simulink model "control_motor"  (R2025a)
settings: Solver=VariableStepAuto  StartTime=0.0  StopTime=10.0  RelTol=1e-3
libraries: fuzblock x1
settings Model: Creator=Bremdows  LastModifiedBy=Bremdows

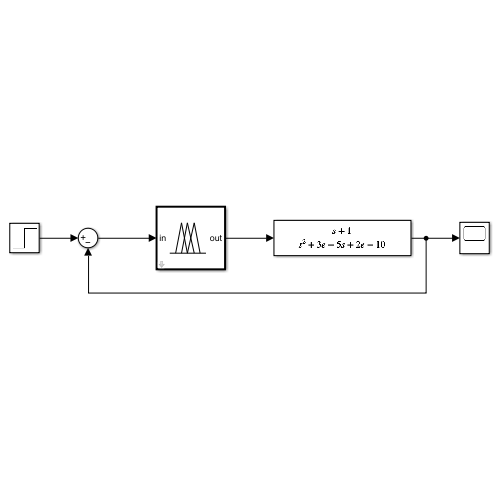
[thumbnail: Simulink's stored preview of the top-level diagram]
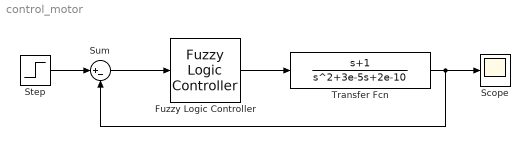
== system control_motor ==
  Fuzzy Logic Controller : fuzblock/Fuzzy Logic  Controller  FIS=faja_motor  OutputSampleNumber=101  DataType=double  UseLookupTable=off  NumBreakpoints=10  FuzzifiedInputs=off  RuleFiringStrengths=off  RuleOutputs=off  AggregatedOutputs=off  SimulateUsing=Interpreted execution  OutOfRangeInputValueMessage=warning  NoRuleFiredMessage=warning  EmptyOutputFuzzySetMessage=warning
  Scope : Scope
  Step : Step  SampleTime=0
  Sum : Sum  Inputs=|+-
  Transfer Fcn : TransferFcn  Numerator=[1 1]  Denominator=[1 3e-5 2e-10]
  wires:
  Step/1 -> Sum/1
  Transfer Fcn/1 -> Sum/2, Scope/1
  Fuzzy Logic Controller/1 -> Transfer Fcn/1
  Sum/1 -> Fuzzy Logic Controller/1
